simulink model "DroneHighLevel"  (R2024a)
settings: Solver=VariableStepAuto  StartTime=0.0  StopTime=10.0  RelTol=1e-3
settings Model: Creator=nabil  LastModifiedBy=nabil

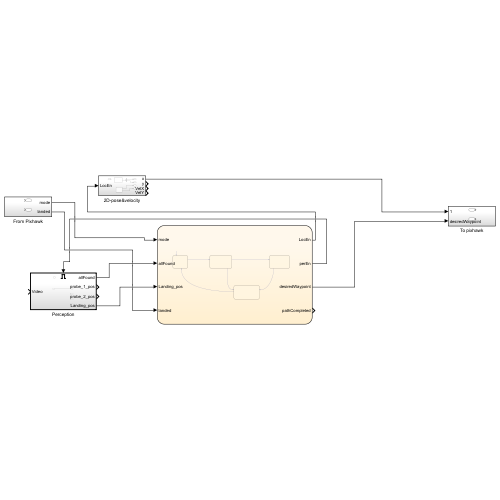
[thumbnail: Simulink's stored preview of the top-level diagram]
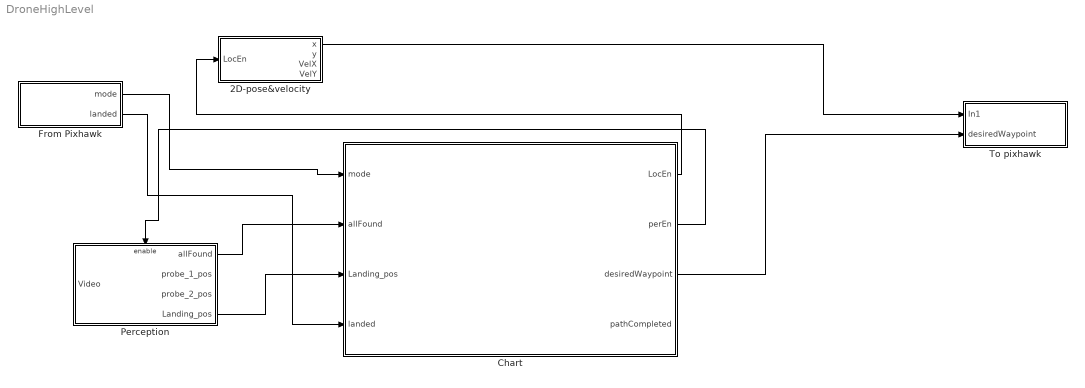
== system DroneHighLevel ==
  2D-pose&velocity : Subsystem
  Chart : Stateflow chart  TreatAsAtomicUnit=on
  From Pixhawk : Subsystem
  Perception : Subsystem
  To pixhawk : Subsystem
  wires:
  From Pixhawk/1(mode) -> Chart/1(mode)
  From Pixhawk/2(landed) -> Chart/4(landed)
  Perception/1(allFound) -> Chart/2(allFound)
  Chart/2(perEn) -> Perception/Enable
  Chart/1(LocEn) -> 2D-pose&velocity/1(LocEn)
  2D-pose&velocity/1(x) -> To pixhawk/1(In1)
  Chart/3(desiredWaypoint) -> To pixhawk/2(desiredWaypoint)
  Perception/4(Landing_pos) -> Chart/3(Landing_pos)

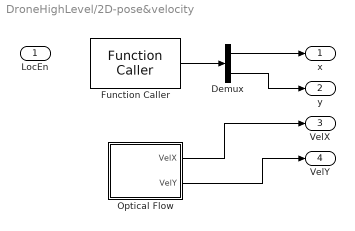
== system DroneHighLevel/2D-pose&velocity ==
  LocEn : Inport
  Demux : Demux  Outputs=2
  Function Caller : FunctionCaller  FunctionPrototype=x = f()  InputArgumentSpecifications=<Enter example>  OutputArgumentSpecifications=<Enter example>
  Optical Flow : Subsystem
  x : Outport
  y : Outport  Port=2
  VelX : Outport  Port=3
  VelY : Outport  Port=4
  wires:
  Optical Flow/1(VelX) -> VelX/1
  Optical Flow/2(VelY) -> VelY/1
  Demux/2 -> y/1
  Demux/1 -> x/1
  Function Caller/1 -> Demux/1

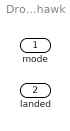
== system DroneHighLevel/From Pixhawk ==
  mode : Outport
  landed : Outport  Port=2

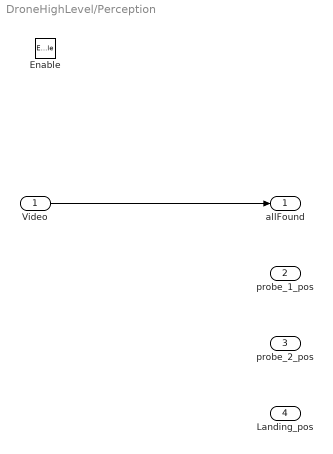
== system DroneHighLevel/Perception ==
  Video : Inport
  Enable : EnablePort
  allFound : Outport
  probe_1_pos : Outport  Port=2
  probe_2_pos : Outport  Port=3
  Landing_pos : Outport  Port=4
  wires:
  Video/1 -> allFound/1

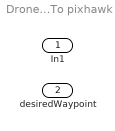
== system DroneHighLevel/To pixhawk ==
  In1 : Inport
  desiredWaypoint : Inport  Port=2

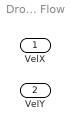
== system DroneHighLevel/2D-pose&velocity/Optical Flow ==
  VelX : Outport
  VelY : Outport  Port=2

== stateflow chart DroneHighLevel/Chart ==
  state DynamicSearch
    entry:
    %%move around the field
  state Idle
    entry:
    perEn=0;
    LocEn=0;
    pathCompleted=0;
  state StaticSearch
    entry:
    perEn=1;
    LocEn=1;
    %%takeoff to desired height
    %%rotate full circle
  state GoToLand
    entry:
    desiredWaypoint=Landing_pos
    %%land
  (default) -> Idle
  StaticSearch -> DynamicSearch [order 1] : after(N,sec)%%set to determine full circle
  Idle -> StaticSearch : [mode==8]%%guided mode
  DynamicSearch -> GoToLand : [allFound==1||PathCompleted==1]
  GoToLand -> Idle : [landed==1]
  StaticSearch -> GoToLand [order 2] : [allFound==1]
  data: PathCompleted local =0; mode input; allFound input; Landing_pos input; landed input; LocEn output; perEn output; N parameter; desiredWaypoint output; pathCompleted output
